simulink model "Jammer_Generator"  (R2024a)
settings: Solver=VariableStepAuto  StartTime=0.0  StopTime=0.005  RelTol=1e-3
InitFcn:
  | % initial_data
undefined symbols (not defined in the file or in its folder): magnitude, model
libraries: simulink x2, commrfcorlib x1, commdigbbndfm2 x1
settings Model: Creator=79327  LastModifiedBy=89778
settings OptimizationCC: ReuseModelBlockBuffer=off
settings RTWCC: GPUComputeCapability=3.5

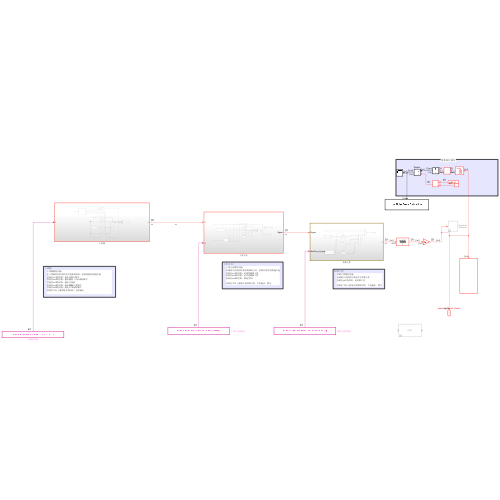
[thumbnail: Simulink's stored preview of the top-level diagram]
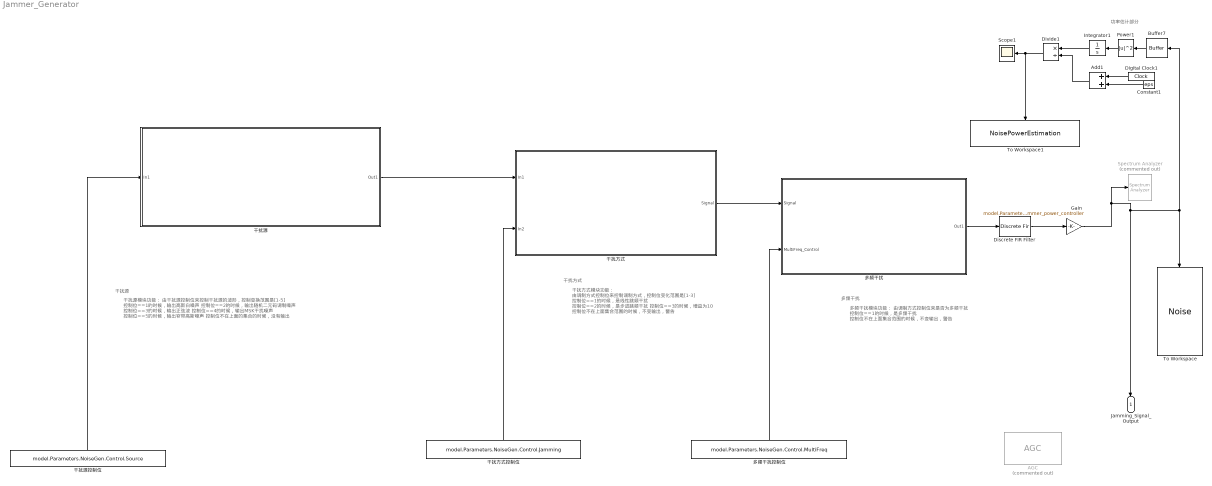
== system Jammer_Generator ==
  note: 功率估计部分
  note: 干扰源模块功能：
      | 由干扰源控制位来控制干扰源的波形，控制变换范围是[1-5]
      | 控制位==1的时候，输出高斯白噪声
      | 控制位==2的时候，输出随机二元码调制噪声
      | 控制位==3的时候，输出正弦波
      | 控制位==4的时候，输出MSK干扰噪声
      | 控制位==5的时候，输出窄带高斯噪声
      | 控制位不在上面的集合的时候，没有输出
  note: 干扰源
  note: 干扰方式
  note: 干扰方式模块功能：
      | 由调制方式控制位来控制调制方式，控制位变化范围是[1-3]
      | 控制位==1的时候，是线性跳频干扰
      | 控制位==2的时候，是步进跳频干扰
      | 控制位==3的时候，增益为10
      |
      | 控制位不在上面集合范围的时候，不变输出，警告
  note: 多频干扰
  note: 多频干扰模块功能：
      | 由调制方式控制位来是否为多频干扰
      | 控制位==1的时候，是多频干扰
      |
      | 控制位不在上面集合范围的时候，不变输出，警告
  AGC : commrfcorlib/AGC  Commented=on  LegacyMode=off  DetectorMethod=Rectifier  LoopMethod=Linear  UpdatePeriod=100  StepSize=0.1  AdaptationStepSize=0.01  DesiredOutputPower=1  AveragingLength=100  MaximumGain=30  MaxPowerGain=60  GainOutputPort=off  InputPowerOutputPort=off  SimulateUsing=Interpreted execution
  Add1 : Sum
  Buffer7 : Buffer  N=1  OutputFrames=off
  Constant1 : Constant  Value=eps  SampleTime=model.Parameters.NoiseGen.NoiseTs
  Digital Clock1 : DigitalClock  SampleTime=model.Parameters.NoiseGen.NoiseTs
  Discrete FIR Filter : DiscreteFir  Coefficients=model.Parameters.NoiseGen.noise_filter_b
  Divide1 : Product  Inputs=*/
  Gain : Gain  Gain=model.Parameters.jammer_power_controller
  Integrator1 : Integrator
  Power1 : Math  Operator=magnitude^2
  Scope1 : Scope
  Spectrum Analyzer : SpectrumAnalyzer  Commented=on  WindowPosition=[162 288 916 450]  SampleRate=340000000  AxesScaling=Manual  Span=340000000  StartFrequency=-170000000  StopFrequency=170000000  AveragingMethod=Exponential  YLimits=[16.792703666476541002,24.095744456486141161]  AllowFFTLengthLessThanSamplesPerUpdate=on
  To Workspace : ToWorkspace  VariableName=Noise  SaveFormat=Timeseries  SampleTime=-1
  To Workspace1 : ToWorkspace  VariableName=NoisePowerEstimation  SaveFormat=Timeseries  SampleTime=-1
  多频干扰 : Subsystem
  多频干扰控制位 : Constant  Value=model.Parameters.NoiseGen.Control.MultiFreq  SampleTime=Inf
  干扰方式 : Subsystem
  干扰方式控制位 : Constant  Value=model.Parameters.NoiseGen.Control.Jamming  SampleTime=Inf
  干扰源 : Subsystem
  干扰源控制位 : Constant  Value=model.Parameters.NoiseGen.Control.Source  SampleTime=Inf
  Jamming_Signal_Output : Outport
  wires:
  干扰方式控制位/1 -> 干扰方式/2(In2)
  干扰源/1(Out1) -> 干扰方式/1(In1)
  干扰源控制位/1 -> 干扰源/1(In1)
  Buffer7/1 -> Power1/1
  Divide1/1 -> Scope1/1, To Workspace1/1
  Integrator1/1 -> Divide1/1
  Digital Clock1/1 -> Add1/1
  Power1/1 -> Integrator1/1
  Add1/1 -> Divide1/2
  Constant1/1 -> Add1/2
  Gain/1 -> Spectrum Analyzer/1, Jamming_Signal_Output/1, Buffer7/1, To Workspace/1
  多频干扰控制位/1 -> 多频干扰/2(MultiFreq_Control)
  干扰方式/1(Signal) -> 多频干扰/1(Signal)
  Discrete FIR Filter/1 -> Gain/1
  多频干扰/1(Out1) -> Discrete FIR Filter/1

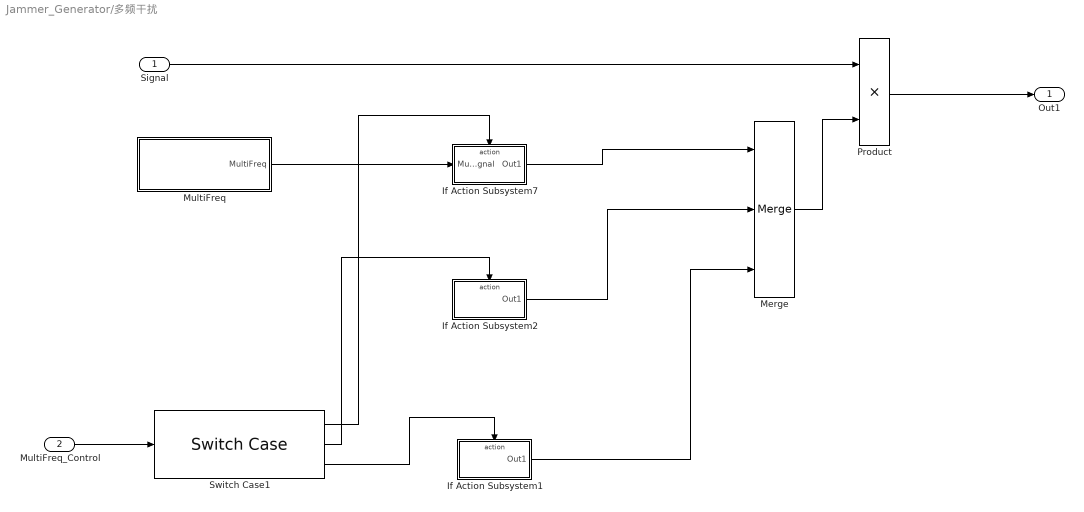
== system Jammer_Generator/多频干扰 ==
  Signal : Inport
  MultiFreq_Control : Inport  Port=2
  If Action Subsystem1 : Subsystem  TreatAsAtomicUnit=on
  If Action Subsystem2 : Subsystem  TreatAsAtomicUnit=on
  If Action Subsystem7 : Subsystem  TreatAsAtomicUnit=on
  Merge : Merge  Inputs=3
  MultiFreq : Subsystem
  Product : Product
  Switch Case1 : SwitchCase  CaseConditions={1,2}
  Out1 : Outport
  wires:
  If Action Subsystem1/1(Out1) -> Merge/3
  Switch Case1/3 -> If Action Subsystem1/Action
  Product/1 -> Out1/1
  If Action Subsystem7/1(Out1) -> Merge/1
  Switch Case1/1 -> If Action Subsystem7/Action
  MultiFreq_Control/1 -> Switch Case1/1
  Merge/1 -> Product/2
  MultiFreq/1(MultiFreq) -> If Action Subsystem7/1(MultiFreqSignal)
  Switch Case1/2 -> If Action Subsystem2/Action
  If Action Subsystem2/1(Out1) -> Merge/2
  Signal/1 -> Product/1

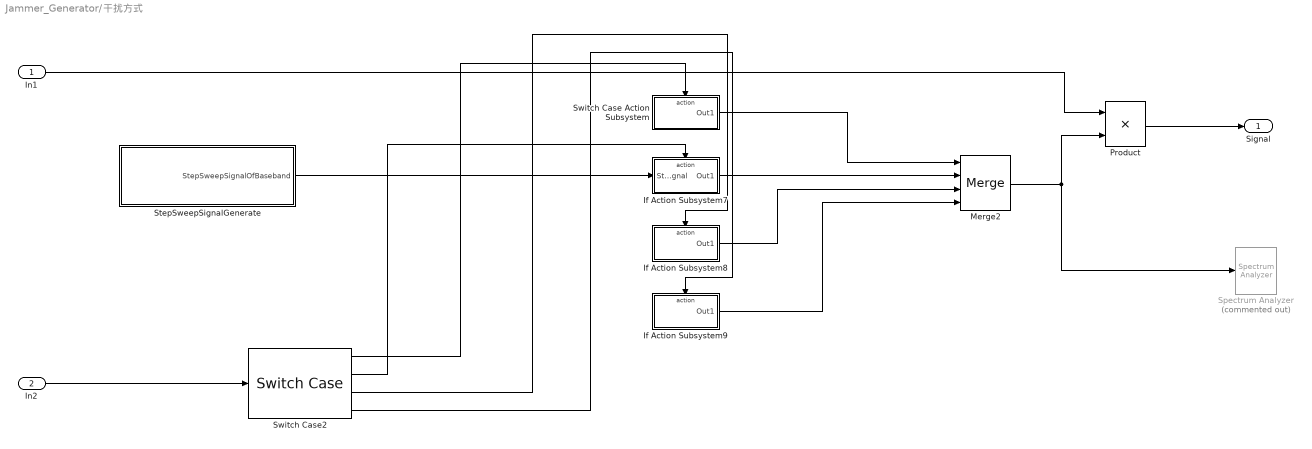
== system Jammer_Generator/干扰方式 ==
  In1 : Inport
  In2 : Inport  Port=2
  If Action Subsystem7 : Subsystem  TreatAsAtomicUnit=on
  If Action Subsystem8 : Subsystem  TreatAsAtomicUnit=on
  If Action Subsystem9 : Subsystem  TreatAsAtomicUnit=on
  Merge2 : Merge  Inputs=4
  Product : Product
  Spectrum Analyzer : SpectrumAnalyzer  Commented=on  WindowPosition=[-1041 199 916 450]  SampleRate=340000000  AxesScaling=Manual  Span=340000000  StartFrequency=-170000000  StopFrequency=170000000  AveragingMethod=Exponential  YLimits=[-55.253534235882824532,34.529267970454846193]  AllowFFTLengthLessThanSamplesPerUpdate=on
  StepSweepSignalGenerate : Subsystem
  Switch Case Action Subsystem : Subsystem  TreatAsAtomicUnit=on
  Switch Case2 : SwitchCase  CaseConditions={1,2,3}
  Signal : Outport
  wires:
  If Action Subsystem9/1(Out1) -> Merge2/4
  Switch Case Action Subsystem/1(Out1) -> Merge2/1
  If Action Subsystem8/1(Out1) -> Merge2/3
  Switch Case2/3 -> If Action Subsystem8/Action
  Switch Case2/1 -> Switch Case Action Subsystem/Action
  Switch Case2/2 -> If Action Subsystem7/Action
  Switch Case2/4 -> If Action Subsystem9/Action
  If Action Subsystem7/1(Out1) -> Merge2/2
  Merge2/1 -> Spectrum Analyzer/1, Product/2
  Product/1 -> Signal/1
  In1/1 -> Product/1
  In2/1 -> Switch Case2/1
  StepSweepSignalGenerate/1(StepSweepSignalOfBaseband) -> If Action Subsystem7/1(StepSweepSignal)

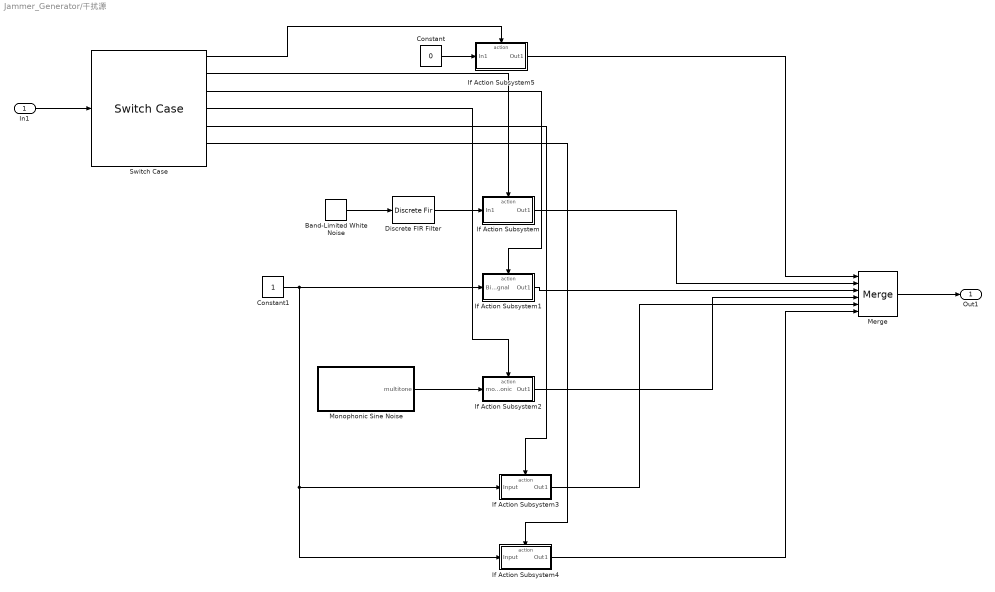
== system Jammer_Generator/干扰源 ==
  In1 : Inport
  Band-Limited White Noise : simulink/Sources/Band-Limited White Noise  Cov=model.Parameters.NoiseGen.GaussPower  Ts=model.Parameters.NoiseGen.NoiseTs  seed=model.Parameters.NoiseGen.GaussSeed
  Constant : Constant  Value=0
  Constant1 : Constant
  Discrete FIR Filter : DiscreteFir  Coefficients=model.Parameters.NoiseGen.pulse_noise_filter_b
  If Action Subsystem : Subsystem  TreatAsAtomicUnit=on
  If Action Subsystem1 : Subsystem  TreatAsAtomicUnit=on
  If Action Subsystem2 : Subsystem  TreatAsAtomicUnit=on
  If Action Subsystem3 : Subsystem  TreatAsAtomicUnit=on
  If Action Subsystem4 : Subsystem  TreatAsAtomicUnit=on
  If Action Subsystem5 : Subsystem  TreatAsAtomicUnit=on
  Merge : Merge  Inputs=6
  Monophonic Sine Noise : Subsystem
  Switch Case : SwitchCase  CaseConditions={0,1,2,3,4,5}
  Out1 : Outport
  wires:
  Switch Case/3 -> If Action Subsystem1/Action
  If Action Subsystem2/1(Out1) -> Merge/4
  Band-Limited White Noise/1 -> Discrete FIR Filter/1
  If Action Subsystem1/1(Out1) -> Merge/3
  Switch Case/4 -> If Action Subsystem2/Action
  Switch Case/2 -> If Action Subsystem/Action
  Merge/1 -> Out1/1
  In1/1 -> Switch Case/1
  Monophonic Sine Noise/1(multitone) -> If Action Subsystem2/1(monophonic)
  Switch Case/5 -> If Action Subsystem3/Action
  If Action Subsystem3/1(Out1) -> Merge/5
  If Action Subsystem/1(Out1) -> Merge/2
  Switch Case/6 -> If Action Subsystem4/Action
  Constant1/1 -> If Action Subsystem4/1(Input), If Action Subsystem3/1(Input), If Action Subsystem1/1(Binary_Random_Signal)
  If Action Subsystem4/1(Out1) -> Merge/6
  Switch Case/1 -> If Action Subsystem5/Action
  If Action Subsystem5/1(Out1) -> Merge/1
  Constant/1 -> If Action Subsystem5/1(In1)
  Discrete FIR Filter/1 -> If Action Subsystem/1(In1)

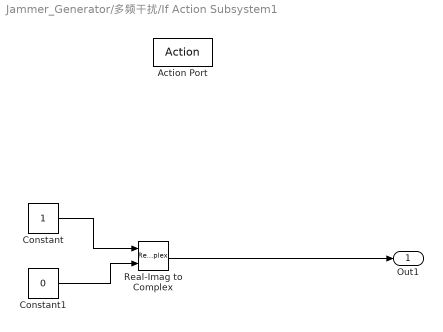
== system Jammer_Generator/多频干扰/If Action Subsystem1 ==
  Action Port : ActionPort  ActionPortLabel=default:
  Constant : Constant
  Constant1 : Constant  Value=0
  Real-Imag to Complex : RealImagToComplex
  Out1 : Outport
  wires:
  Constant/1 -> Real-Imag to Complex/1
  Real-Imag to Complex/1 -> Out1/1
  Constant1/1 -> Real-Imag to Complex/2

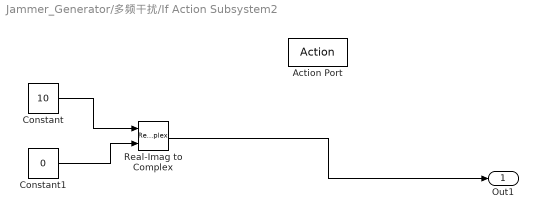
== system Jammer_Generator/多频干扰/If Action Subsystem2 ==
  Action Port : ActionPort  ActionPortLabel=case [ 2 ]:
  Constant : Constant  Value=10
  Constant1 : Constant  Value=0
  Real-Imag to Complex : RealImagToComplex
  Out1 : Outport
  wires:
  Real-Imag to Complex/1 -> Out1/1
  Constant1/1 -> Real-Imag to Complex/2
  Constant/1 -> Real-Imag to Complex/1

== system Jammer_Generator/多频干扰/If Action Subsystem7 ==
  MultiFreqSignal : Inport
  Action Port : ActionPort  ActionPortLabel=case [ 1 ]:
  Out1 : Outport
  wires:
  MultiFreqSignal/1 -> Out1/1

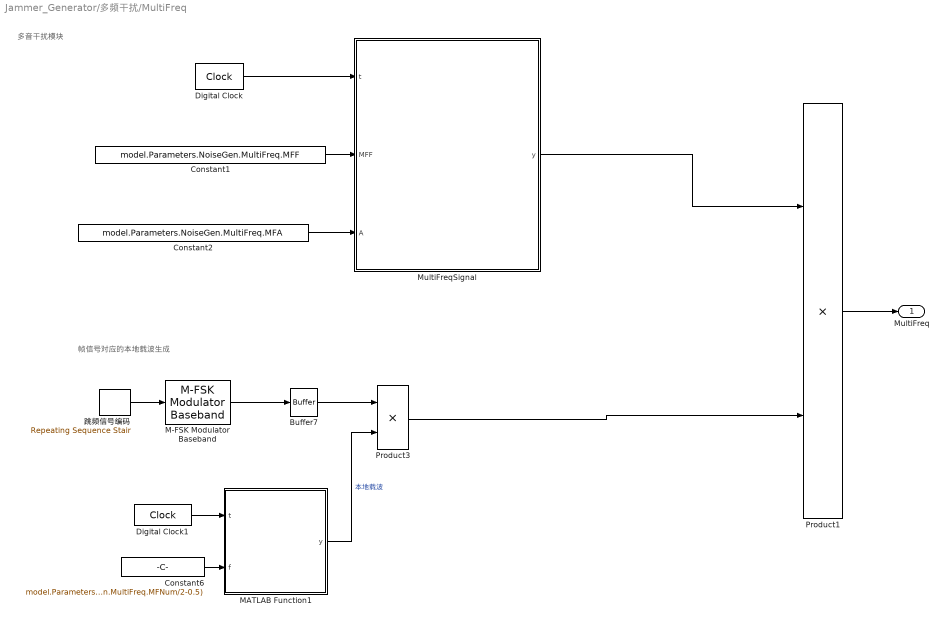
== system Jammer_Generator/多频干扰/MultiFreq ==
  note: 多音干扰模块
  note: 帧信号对应的本地载波生成
  Buffer7 : Buffer  N=1  OutputFrames=off
  Constant1 : Constant  Value=model.Parameters.NoiseGen.MultiFreq.MFF
  Constant2 : Constant  Value=model.Parameters.NoiseGen.MultiFreq.MFA
  Constant6 : Constant  Value=model.Parameters.NoiseGen.MultiFreq.MFDistance*(model.Parameters.NoiseGen.MultiFreq.MFNum/2-0.5)
  Digital Clock : DigitalClock  SampleTime=model.Parameters.NoiseGen.NoiseTs
  Digital Clock1 : DigitalClock  SampleTime=model.Parameters.NoiseGen.NoiseTs
  M-FSK Modulator Baseband : commdigbbndfm2/M-FSK Modulator Baseband  M=model.Parameters.NoiseGen.MultiFreq.MFNum  InType=Integer  Enc=Binary  freqSep=model.Parameters.NoiseGen.MultiFreq.MFDistance  phaseType=Continuous  numSamp=ceil(model.Parameters.NoiseGen.MultiFreq.MFTime/model.Parameters.NoiseGen.NoiseTs)  RateOptions=Enforce single-rate processing  outDataType=double
  MATLAB Function1 : MATLAB Function  InitFcn=|  TreatAsAtomicUnit=on
      | f_chirp_min=4.8e6;
      | f_chirp_max=5.2e6;
      | T_chirp=4e-4;
  MultiFreqSignal : MATLAB Function  TreatAsAtomicUnit=on
  Product1 : Product
  Product3 : Product
  跳频信号编码 : simulink/Sources/Repeating Sequence Stair  OutValues=model.Parameters.NoiseGen.MultiFreq.MFSequence  tsamp=model.Parameters.NoiseGen.NoiseTs*ceil(model.Parameters.NoiseGen.MultiFreq.MFTime/model.Parameters.NoiseGen.NoiseTs)  OutMin=[]  OutMax=[]  OutDataTypeStr=double  OutputDataTypeScalingMode=double  OutDataType=fixdt(0,8)  ConRadixGroup=Best Precision: Vector-wise  OutScaling=2^-12
  MultiFreq : Outport
  wires:
  Constant1/1 -> MultiFreqSignal/2(MFF)
  MultiFreqSignal/1(y) -> Product1/1
  Product1/1 -> MultiFreq/1
  Digital Clock/1 -> MultiFreqSignal/1(t)
  Constant2/1 -> MultiFreqSignal/3(A)
  Digital Clock1/1 -> MATLAB Function1/1(t)
  Buffer7/1 -> Product3/1
  跳频信号编码/1 -> M-FSK Modulator Baseband/1
  M-FSK Modulator Baseband/1 -> Buffer7/1
  MATLAB Function1/1(y) -> Product3/2  "本地载波"
  Constant6/1 -> MATLAB Function1/2(f)
  Product3/1 -> Product1/2

== system Jammer_Generator/干扰方式/If Action Subsystem7 ==
  StepSweepSignal : Inport
  Action Port : ActionPort  ActionPortLabel=case [ 2 ]:
  Out1 : Outport
  wires:
  StepSweepSignal/1 -> Out1/1

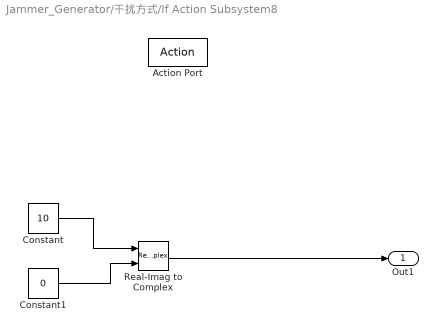
== system Jammer_Generator/干扰方式/If Action Subsystem8 ==
  Action Port : ActionPort  ActionPortLabel=case [ 3 ]:
  Constant : Constant  Value=10
  Constant1 : Constant  Value=0
  Real-Imag to Complex : RealImagToComplex
  Out1 : Outport
  wires:
  Constant/1 -> Real-Imag to Complex/1
  Real-Imag to Complex/1 -> Out1/1
  Constant1/1 -> Real-Imag to Complex/2

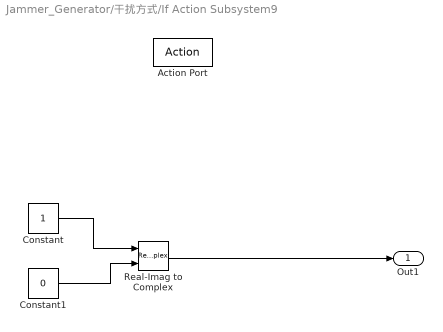
== system Jammer_Generator/干扰方式/If Action Subsystem9 ==
  Action Port : ActionPort  ActionPortLabel=default:
  Constant : Constant
  Constant1 : Constant  Value=0
  Real-Imag to Complex : RealImagToComplex
  Out1 : Outport
  wires:
  Constant/1 -> Real-Imag to Complex/1
  Real-Imag to Complex/1 -> Out1/1
  Constant1/1 -> Real-Imag to Complex/2

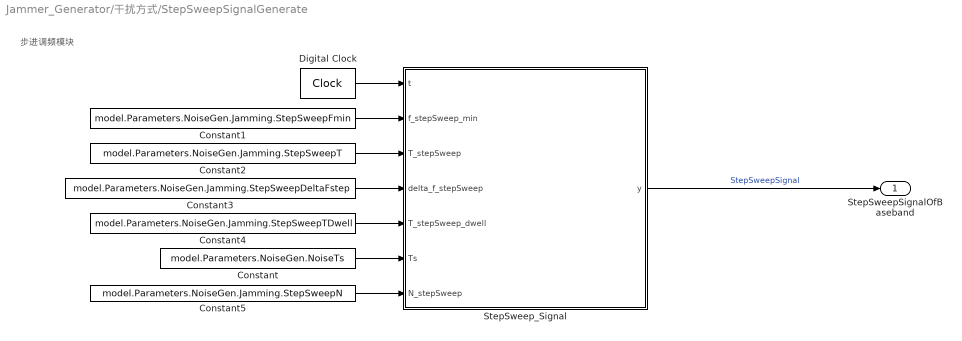
== system Jammer_Generator/干扰方式/StepSweepSignalGenerate ==
  note: 步进调频模块
  Constant : Constant  Value=model.Parameters.NoiseGen.NoiseTs
  Constant1 : Constant  Value=model.Parameters.NoiseGen.Jamming.StepSweepFmin
  Constant2 : Constant  Value=model.Parameters.NoiseGen.Jamming.StepSweepT
  Constant3 : Constant  Value=model.Parameters.NoiseGen.Jamming.StepSweepDeltaFstep
  Constant4 : Constant  Value=model.Parameters.NoiseGen.Jamming.StepSweepTDwell
  Constant5 : Constant  Value=model.Parameters.NoiseGen.Jamming.StepSweepN
  Digital Clock : DigitalClock  SampleTime=model.Parameters.NoiseGen.NoiseTs
  StepSweep_Signal : MATLAB Function  TreatAsAtomicUnit=on
  StepSweepSignalOfBaseband : Outport
  wires:
  Digital Clock/1 -> StepSweep_Signal/1(t)
  StepSweep_Signal/1(y) -> StepSweepSignalOfBaseband/1  "StepSweepSignal"
  Constant/1 -> StepSweep_Signal/6(Ts)
  Constant1/1 -> StepSweep_Signal/2(f_stepSweep_min)
  Constant2/1 -> StepSweep_Signal/3(T_stepSweep)
  Constant3/1 -> StepSweep_Signal/4(delta_f_stepSweep)
  Constant4/1 -> StepSweep_Signal/5(T_stepSweep_dwell)
  Constant5/1 -> StepSweep_Signal/7(N_stepSweep)

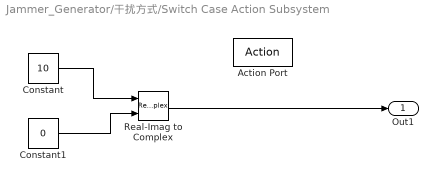
== system Jammer_Generator/干扰方式/Switch Case Action Subsystem ==
  Action Port : ActionPort  ActionPortLabel=case [ 1 ]:
  Constant : Constant  Value=10
  Constant1 : Constant  Value=0
  Real-Imag to Complex : RealImagToComplex
  Out1 : Outport
  wires:
  Real-Imag to Complex/1 -> Out1/1
  Constant1/1 -> Real-Imag to Complex/2
  Constant/1 -> Real-Imag to Complex/1

== system Jammer_Generator/干扰源/If Action Subsystem ==
  In1 : Inport
  Action Port : ActionPort  ActionPortLabel=case [ 1 ]:
  Out1 : Outport
  wires:
  In1/1 -> Out1/1

== system Jammer_Generator/干扰源/If Action Subsystem1 ==
  Binary_Random_Signal : Inport
  Action Port : ActionPort  ActionPortLabel=case [ 2 ]:
  Out1 : Outport
  wires:
  Binary_Random_Signal/1 -> Out1/1

== system Jammer_Generator/干扰源/If Action Subsystem2 ==
  monophonic : Inport
  Action Port : ActionPort  ActionPortLabel=case [ 3 ]:
  Out1 : Outport
  wires:
  monophonic/1 -> Out1/1

== system Jammer_Generator/干扰源/If Action Subsystem3 ==
  Input : Inport
  Action Port : ActionPort  ActionPortLabel=case [ 4 ]:
  Out1 : Outport
  wires:
  Input/1 -> Out1/1

== system Jammer_Generator/干扰源/If Action Subsystem4 ==
  Input : Inport
  Action Port : ActionPort  ActionPortLabel=case [ 5 ]:
  Out1 : Outport
  wires:
  Input/1 -> Out1/1

== system Jammer_Generator/干扰源/If Action Subsystem5 ==
  In1 : Inport
  Action Port : ActionPort  ActionPortLabel=case [ 0 ]:
  Out1 : Outport
  wires:
  In1/1 -> Out1/1

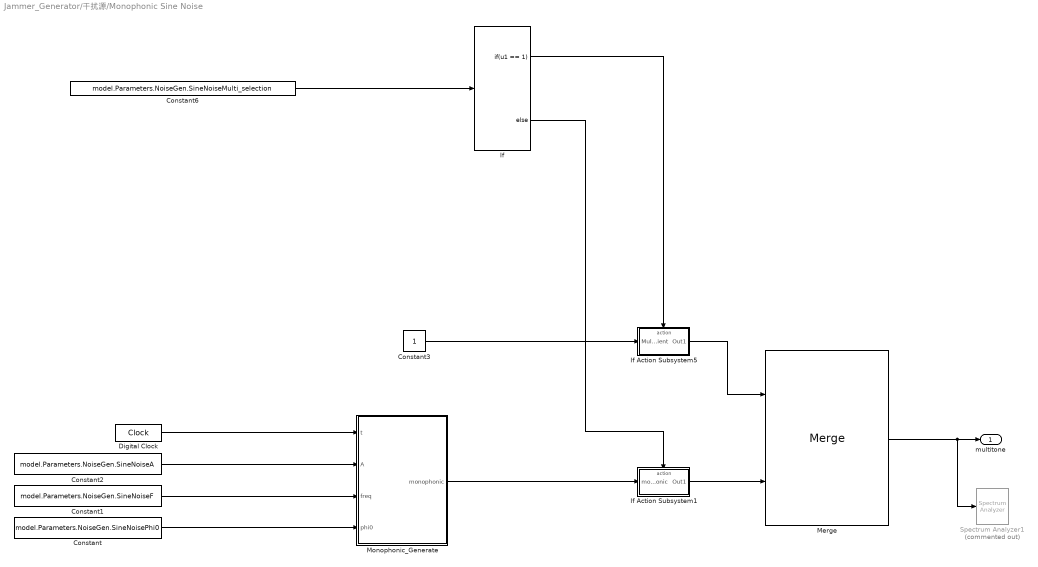
== system Jammer_Generator/干扰源/Monophonic Sine Noise ==
  Constant : Constant  Value=model.Parameters.NoiseGen.SineNoisePhi0
  Constant1 : Constant  Value=model.Parameters.NoiseGen.SineNoiseF
  Constant2 : Constant  Value=model.Parameters.NoiseGen.SineNoiseA
  Constant3 : Constant
  Constant6 : Constant  Value=model.Parameters.NoiseGen.SineNoiseMulti_selection
  Digital Clock : DigitalClock  SampleTime=model.Parameters.NoiseGen.NoiseTs
  If : If  IfExpression=u1 == 1
  If Action Subsystem1 : Subsystem  TreatAsAtomicUnit=on
  If Action Subsystem5 : Subsystem  TreatAsAtomicUnit=on
  Merge : Merge
  Monophonic_Generate : MATLAB Function  TreatAsAtomicUnit=on
  Spectrum Analyzer1 : SpectrumAnalyzer  Commented=on  WindowPosition=[-1168 236 916 450]  SampleRate=340000000  AxesScaling=Manual  Span=340000000  StartFrequency=-170000000  StopFrequency=170000000  AveragingMethod=Exponential  YLimits=[-88.119268432802542179,31.5056137623361181]  AllowFFTLengthLessThanSamplesPerUpdate=on
  multitone : Outport
  wires:
  Digital Clock/1 -> Monophonic_Generate/1(t)
  Constant/1 -> Monophonic_Generate/4(phi0)
  Constant2/1 -> Monophonic_Generate/2(A)
  Constant1/1 -> Monophonic_Generate/3(freq)
  Merge/1 -> Spectrum Analyzer1/1, multitone/1
  Constant6/1 -> If/1
  If/1 -> If Action Subsystem5/Action
  If/2 -> If Action Subsystem1/Action
  If Action Subsystem5/1(Out1) -> Merge/1
  Monophonic_Generate/1(monophonic) -> If Action Subsystem1/1(monophonic)
  If Action Subsystem1/1(Out1) -> Merge/2
  Constant3/1 -> If Action Subsystem5/1(Multitone_multiplicative_coefficient)

== system Jammer_Generator/干扰源/Monophonic Sine Noise/If Action Subsystem1 ==
  monophonic : Inport
  Action Port : ActionPort  ActionPortLabel=else
  Out1 : Outport
  wires:
  monophonic/1 -> Out1/1

== system Jammer_Generator/干扰源/Monophonic Sine Noise/If Action Subsystem5 ==
  Multitone_multiplicative_coefficient : Inport
  Action Port : ActionPort  ActionPortLabel=if(u1 == 1)
  Out1 : Outport
  wires:
  Multitone_multiplicative_coefficient/1 -> Out1/1

== matlab function Jammer_Generator/干扰源/Monophonic Sine Noise/Monophonic_Generate ==
  data: t input; A input; freq input; monophonic output; phi0 input
function monophonic = MonophonicGenerate(t, A, freq, phi0)
    monophonic = A * cos(2*pi*freq*t+phi0);
end

== matlab function Jammer_Generator/干扰方式/StepSweepSignalGenerate/StepSweep_Signal ==
  data: y output; t input; f_stepSweep_min input; T_stepSweep input; delta_f_stepSweep input; T_stepSweep_dwell input; Ts input; N_stepSweep input
function y  = StepSweep(t, f_stepSweep_min, T_stepSweep, delta_f_stepSweep, T_stepSweep_dwell, Ts, N_stepSweep)
    a = mod(t,T_stepSweep) + Ts/10000;
    b = fix(a/T_stepSweep_dwell);
    if b == N_stepSweep
        b = N_stepSweep - 1;
    end
    f = (f_stepSweep_min + b*delta_f_stepSweep);
    y = exp(1i*2*pi*f*t);
end

== matlab function Jammer_Generator/多频干扰/MultiFreq/MATLAB Function1 ==
  data: y output; t input; f input
% function y = carrierGenerator(t)
%     fc = 5e6;
%     y = exp(1i*2*pi*fc*t);

function y = carrierGenerator(t, f)
    y = exp(1i*2*pi*f*t);
end

== matlab function Jammer_Generator/多频干扰/MultiFreq/MultiFreqSignal ==
  data: y output; t input; MFF input; A input
function y  = MultiFreqSignal(t, MFF,A)
    % MFF表示输入的多频信号的频率与原信号的频率间隔
    % t表示采样时间
    % Signal表示需要被多频调制的原信号
    % A表示对应幅值
    % Phi0表示对应相位
    N = length(MFF); 
    MultitoneSignal =complex(zeros(N,1));
    for num1=1:N
        MultitoneSignal(num1) = A(num1).*exp(1j*(2*pi.*MFF(num1)*t));
    end
    y = sum(MultitoneSignal,"all");
end
